simulink model "DynamicIntegration_TestModel"  (R2014a)
settings: Solver=ode3  StartTime=0.0  StopTime=10.0  FixedStep=0.01  RelTol=1e-3
InitFcn:
  | data_parametric_model
undefined symbols (not defined in the file or in its folder): cog_motor, dry_motor_weight, dry_rocket_cog, dry_rocket_mass, dry_rocket_moi, dry_rocket_weight, length_motor, mass_flow_rate, wet_motor_mass, wet_motor_weight
libraries: rocket_dynamic_data_library x4
settings Model: Creator=scorpii  LastModifiedBy=scorpii

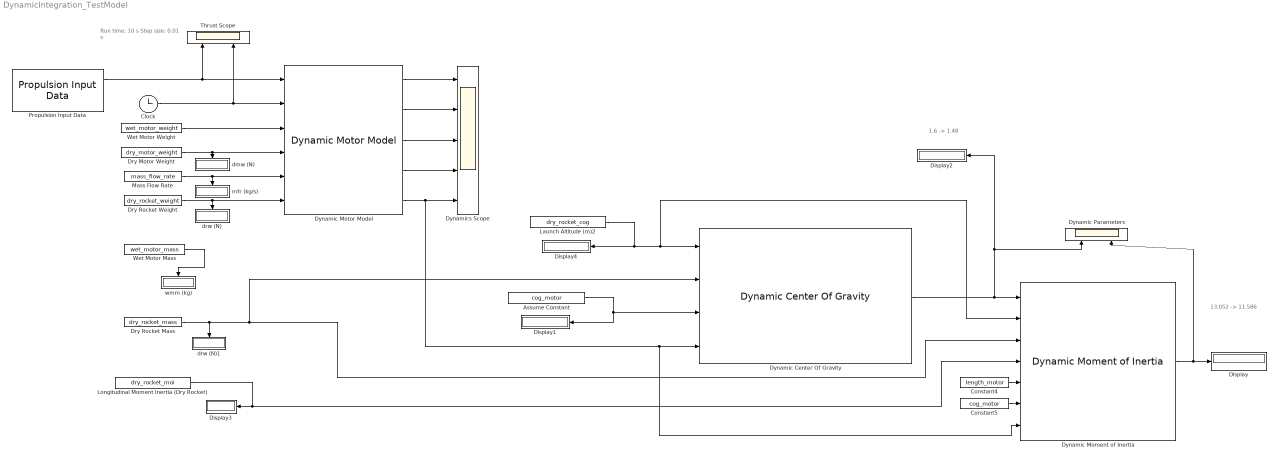
== system DynamicIntegration_TestModel ==
  note: Run time: 10 s
      | Step size: 0.01 s
  note: 13.052 -> 11.586
  note: 1.6 -> 1.48
  Assume Constant : Constant  Value=cog_motor
  Clock : Clock
  Constant4 : Constant  Value=length_motor
  Constant5 : Constant  Value=cog_motor
  Display{,1..4} (5 alike) : Display
  Dry Motor Weight : Constant  Value=dry_motor_weight
  Dry Rocket Mass : Constant  Value=dry_rocket_mass
  Dry Rocket Weight : Constant  Value=dry_rocket_weight
  Dynamic Center Of Gravity : rocket_dynamic_data_library/Dynamic Center Of Gravity
  Dynamic Moment of Inertia : rocket_dynamic_data_library/Dynamic Moment of Inertia
  Dynamic Motor Model : rocket_dynamic_data_library/Dynamic Motor Model
  Dynamic Parameters : Scope  NumInputPorts=2
      settings: YMin=126.243~1238.44  YMax=139.531~1368.8
  Dynamics Scope : Scope  NumInputPorts=5
      settings: YMin=126.243~1238.44~774.486~-5~-5  YMax=139.531~1368.8~856.01~5~5
  Launch Altitude (m)2 : Constant  Value=dry_rocket_cog
  Longitudinal Moment Inertia (Dry Rocket) : Constant  Value=dry_rocket_moi
  Mass Flow Rate : Constant  Value=mass_flow_rate
  Propulsion Input Data : rocket_dynamic_data_library/Propulsion Input Data
  Thrust Scope : Scope  NumInputPorts=2
      settings: YMin=126.243~1238.44  YMax=139.531~1368.8  SaveName=ScopeData2
  Wet Motor Mass : Constant  Value=wet_motor_mass
  Wet Motor Weight : Constant  Value=wet_motor_weight
  dmw (N) : Display
  drw (N) : Display
  drw (N)1 : Display
  mfr (kg/s) : Display
  wmm (kg) : Display
  wires:
  Launch Altitude (m)2/1 -> Dynamic Center Of Gravity/1, Dynamic Moment of Inertia/2, Display4/1
  Assume Constant/1 -> Dynamic Center Of Gravity/3, Display1/1
  Dynamic Center Of Gravity/1 -> Display2/1, Dynamic Parameters/1, Dynamic Moment of Inertia/1
  Dry Rocket Weight/1 -> Dynamic Motor Model/6, drw (N)/1
  Longitudinal Moment Inertia (Dry Rocket)/1 -> Dynamic Moment of Inertia/4, Display3/1
  Constant4/1 -> Dynamic Moment of Inertia/5
  Constant5/1 -> Dynamic Moment of Inertia/6
  Dynamic Moment of Inertia/1 -> Dynamic Parameters/2, Display/1
  Clock/1 -> Dynamic Motor Model/2, Thrust Scope/2
  Propulsion Input Data/1 -> Dynamic Motor Model/1, Thrust Scope/1
  Dry Motor Weight/1 -> Dynamic Motor Model/4, dmw (N)/1
  Mass Flow Rate/1 -> Dynamic Motor Model/5, mfr (kg/s)/1
  Wet Motor Mass/1 -> wmm (kg)/1
  Dynamic Motor Model/4 -> Dynamics Scope/4
  Dynamic Motor Model/5 -> Dynamic Moment of Inertia/7, Dynamic Center Of Gravity/4, Dynamics Scope/5
  Wet Motor Weight/1 -> Dynamic Motor Model/3
  Dynamic Motor Model/1 -> Dynamics Scope/1
  Dynamic Motor Model/2 -> Dynamics Scope/2
  Dynamic Motor Model/3 -> Dynamics Scope/3
  Dry Rocket Mass/1 -> drw (N)1/1, Dynamic Center Of Gravity/2, Dynamic Moment of Inertia/3
